simulink model "exercicio2aula"  (R2022a)
settings: Solver=VariableStepAuto  StartTime=0.0  StopTime=10.0  RelTol=1e-3
settings Model: Creator=a2150336  LastModifiedBy=a2150336

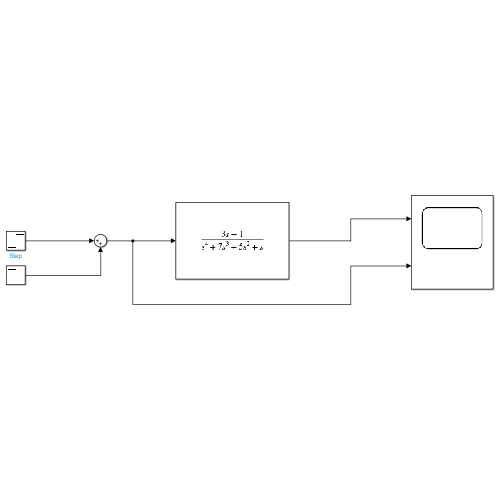
[thumbnail: Simulink's stored preview of the top-level diagram]
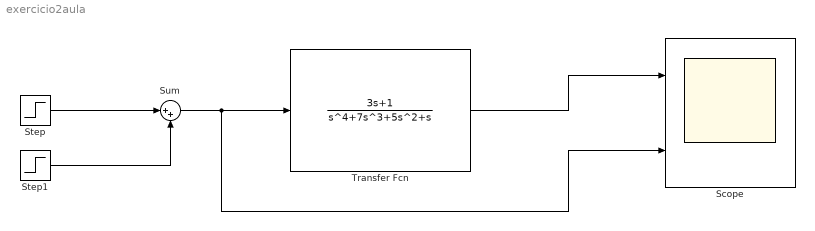
== system exercicio2aula ==
  Scope : Scope  NumInputPorts=2
  Step : Step  SampleTime=0
  Step1 : Step  Time=2  After=-1  SampleTime=0
  Sum : Sum  Inputs=|++
  Transfer Fcn : TransferFcn  Numerator=[0 0 0 3 1]  Denominator=[1 7 5 1 0]
  wires:
  Transfer Fcn/1 -> Scope/1
  Sum/1 -> Scope/2, Transfer Fcn/1
  Step/1 -> Sum/1
  Step1/1 -> Sum/2
